simulink model "StateTransition"  (R2020a)
settings: Solver=FixedStepDiscrete  StartTime=0.0  StopTime=10.0  FixedStep=1.0  RelTol=1e-3
libraries: simulink x2
settings Model: Creator=ashok  LastModifiedBy=ashok

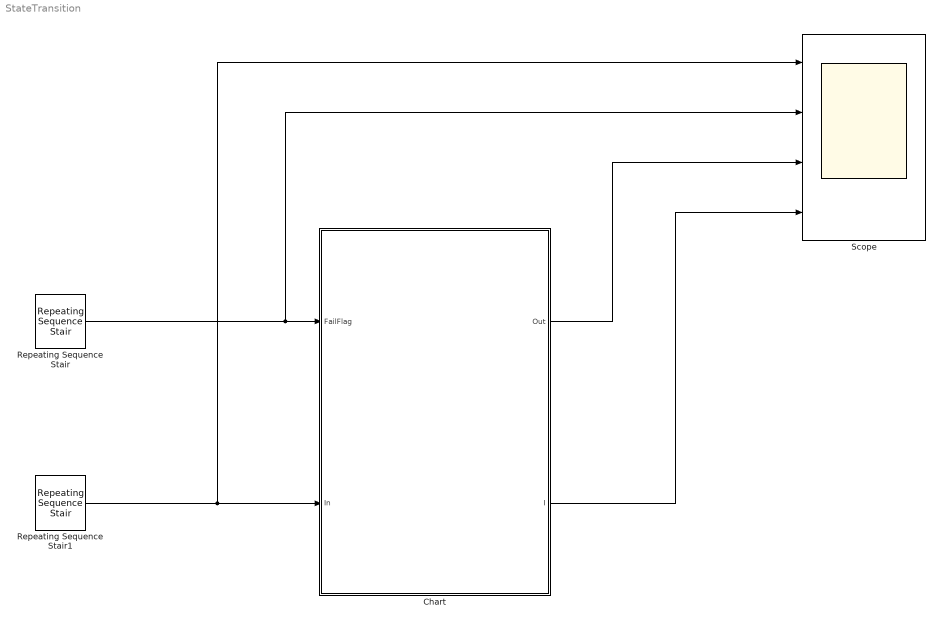
== system StateTransition ==
  Chart : Stateflow chart  TreatAsAtomicUnit=on
  Repeating Sequence Stair : simulink/Sources/Repeating Sequence Stair  OutValues=[0 1].'  tsamp=-1  OutMin=[]  OutMax=[]  OutDataTypeStr=double  OutputDataTypeScalingMode=double  OutDataType=fixdt(0,8)  ConRadixGroup=Best Precision: Vector-wise  OutScaling=2^-12
  Repeating Sequence Stair1 : simulink/Sources/Repeating Sequence Stair  OutValues=[3 1 4 2 1].'  tsamp=-1  OutMin=[]  OutMax=[]  OutDataTypeStr=double  OutputDataTypeScalingMode=double  OutDataType=fixdt(0,8)  ConRadixGroup=Best Precision: Vector-wise  OutScaling=2^-12
  Scope : Scope  NumInputPorts=4
  wires:
  Repeating Sequence Stair/1 -> Scope/2, Chart/1(FailFlag)
  Repeating Sequence Stair1/1 -> Scope/1, Chart/2(In)
  Chart/2(I) -> Scope/4
  Chart/1(Out) -> Scope/3

== stateflow chart StateTransition/Chart ==
  state Normal
    en:
    Out = In;
    du:
    Out = In;
  state Fail
    en:
    I = 1;
    Out = 0;
    du:
    I = I+1;
  (default) -> Normal
  Normal -> Fail : [FailFlag == 1]
  Fail -> Normal [order 2] : [I == 5]
  Fail -> Fail [order 1] : [FailFlag == 1]
  data: FailFlag input; In input; Out output; I output
